simulink model "Nghich_luu2"  (R2019a)
settings: Solver=VariableStepAuto  StartTime=0.0  StopTime=10.0  RelTol=1e-3
libraries: powerlib x17, powerlib_meascontrol x2
settings Model: Creator=Admin  LastModifiedBy=Admin

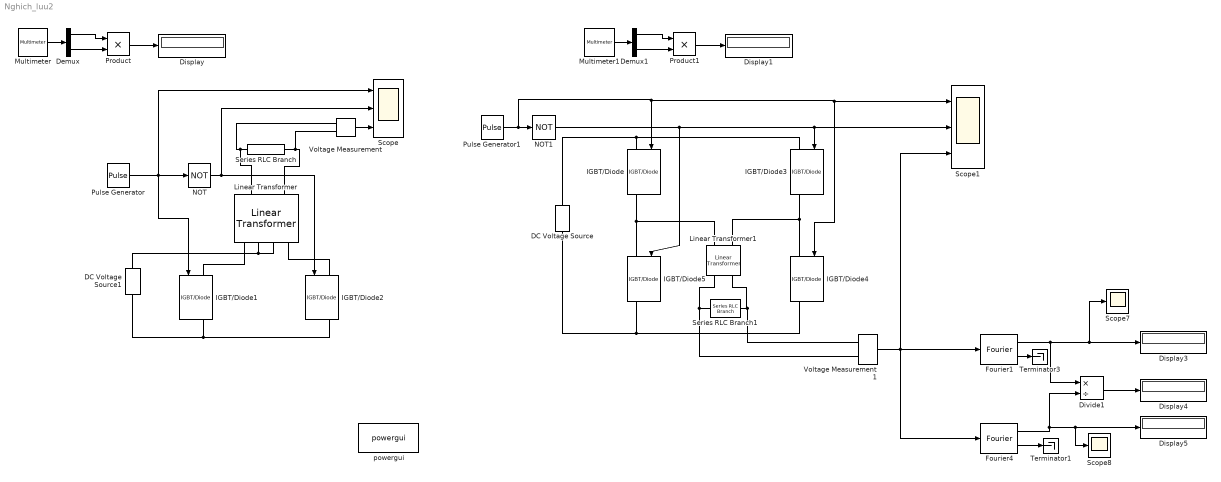
== system Nghich_luu2 ==
  DC Voltage Source : powerlib/Electrical Sources/DC Voltage Source  Amplitude=100  Measurements=None
      settings: SourceProductName=Simscape Electrical
  DC Voltage Source1 : powerlib/Electrical Sources/DC Voltage Source  Amplitude=12  Measurements=None
      settings: SourceProductName=Simscape Electrical
  Demux : Demux  Outputs=2
  Demux1 : Demux  Outputs=2
  Display{,1,3..5} (5 alike) : Display
  Divide1 : Product  Inputs=*/
  Fourier1 : powerlib_meascontrol/Measurements/Fourier  Freq=50  n=1  InInit=[0, 0]  Ts=0
      settings: SourceProductName=Simscape Electrical
  Fourier4 : powerlib_meascontrol/Measurements/Fourier  Freq=50  n=0  InInit=[0, 0]  Ts=0
      settings: SourceProductName=Simscape Electrical
  IGBT/Diode{,1..5} (6 alike) : powerlib/Power Electronics/IGBT//Diode  Ron=1e-3  Rs=1e5  Cs=inf  Measurements=on
      settings: SourceProductName=Simscape Electrical
  Linear Transformer : powerlib/Elements/Linear Transformer  UNITS=SI  NominalPower=[200 50]  winding1=[220 0 0]  winding2=[12 0 0]  ThreeWindings=on  winding3=[12 0 0]  RmLm=[1.21e+05 385.15]  Measurements=None  DataType=on
      settings: SourceProductName=Simscape Electrical
  Linear Transformer1 : powerlib/Elements/Linear Transformer  UNITS=SI  NominalPower=[ 300 50 ]  winding1=[12 0.02 0]  winding2=[220 0.05 0]  ThreeWindings=off  winding3=[3.15e+05 0.7938 0.084224]  RmLm=[inf inf]  Measurements=None  DataType=on
      settings: SourceProductName=Simscape Electrical
  Multimeter : powerlib/Measurements/Multimeter  PhasorSimulation=off  OutputType=Complex  sel=[1 3]  L=4  Gain=[1 1]  yselected={'Ub: Series RLC Branch','Ib: Series RLC Branch'};  PSBOutputType=1  PSBequivalent=0  AxesSetting=[0,0.1,-100,100]  Display=0  SavedBlockNames=-11
      settings: SourceProductName=Simscape Electrical
  Multimeter1 : powerlib/Measurements/Multimeter  PhasorSimulation=off  OutputType=Complex  sel=[2 4]  L=4  Gain=[1 1]  yselected={'Ub: Series RLC Branch1','Ib: Series RLC Branch1'};  PSBOutputType=1  PSBequivalent=0  AxesSetting=[0,0.1,-100,100]  Display=0  SavedBlockNames=-11
      settings: SourceProductName=Simscape Electrical
  NOT : Logic  Operator=NOT  IconShape=distinctive  AllPortsSameDT=off  OutDataTypeStr=boolean
  NOT1 : Logic  Operator=NOT  IconShape=distinctive  AllPortsSameDT=off  OutDataTypeStr=boolean
  Product : Product
  Product1 : Product
  Pulse Generator : DiscretePulseGenerator  PulseType=Time based  Period=0.02  PulseWidth=50
  Pulse Generator1 : DiscretePulseGenerator  PulseType=Time based  Period=0.02  PulseWidth=50
  Scope : Scope  NumInputPorts=3
  Scope1 : Scope  NumInputPorts=3
  Scope7 : Scope
  Scope8 : Scope
  Series RLC Branch : powerlib/Elements/Series RLC Branch  LConnTagsString=__new0  RConnTagsString=__new0  BranchType=R  Resistance=200  Inductance=1e-3  SetiL0=off  InitialCurrent=0  Capacitance=1e-6  Setx0=off  InitialVoltage=0  Measurements=Branch voltage and current
      settings: SourceProductName=Simscape Electrical
  Series RLC Branch1 : powerlib/Elements/Series RLC Branch  LConnTagsString=__new0  RConnTagsString=__new0  BranchType=R  Resistance=1.1  Inductance=1e-3  SetiL0=off  InitialCurrent=0  Capacitance=1e-6  Setx0=off  InitialVoltage=0  Measurements=Branch voltage and current
      settings: SourceProductName=Simscape Electrical
  Terminator1 : Terminator
  Terminator3 : Terminator
  Voltage Measurement : powerlib/Measurements/Voltage Measurement  PhasorSimulation=off  OutputType=Complex  PSBequivalent=0
      settings: SourceProductName=Simscape Electrical
  Voltage Measurement1 : powerlib/Measurements/Voltage Measurement  PhasorSimulation=off  OutputType=Complex  PSBequivalent=0
      settings: SourceProductName=Simscape Electrical
  powergui : powerlib/powergui  Priority=1  SimulationMode=Continuous  SampleTime=50e-6  frequency=60  Iterations=50  frequencyindice=0  Pbase=100e6  ErrMax=1e-4  UnitsV=kV  UnitsW=MW  buscounter=0  FunctionMessages=off  echomessages=off  EnableUseOfTLC=off  CurrentSourceSwitches=off  DisableSnubberDevices=off  DisableRonSwitches=off  DisableVfSwitches=off  DisplayEquations=off  AutomaticDiscreteSolvers=off  SolverType=Tustin/Backward Euler (TBE)  Interpol=off  ExternalGateDelay=off  methode=off  Ts=100  x0status=blocks  SPID=on  SwTol=0  HookPort=off  NonlinearTolerance=0  nMaxIteration=15  ContinueOnMaxIteration=off  RestoreLinks=warning  ResistiveCurrentMeasurement=off  Frange=[0:2:500]  Ylog=off  Xlog=on  ShowGrid=off  save=off  variable=ZData  structure=0  ZoomFFT=off  StartTime=0.0  cycles=1  DisplayStyle=1  fundamental=60  FreqAxis=off  MaxFrequency=1000  frequencyindicesteady=1  RmsSteady=1  display=off
      settings: SourceProductName=Simscape Electrical
  wires:
  Voltage Measurement/1 -> Scope/3
  Pulse Generator/1 -> Scope/1, IGBT/Diode1/1, NOT/1
  NOT/1 -> Scope/2, IGBT/Diode2/1
  Pulse Generator1/1 -> IGBT/Diode4/1, Scope1/1, IGBT/Diode/1, NOT1/1
  NOT1/1 -> IGBT/Diode5/1, IGBT/Diode3/1, Scope1/2
  Fourier1/2 -> Terminator3/1
  Divide1/1 -> Display4/1
  Fourier1/1 -> Divide1/1, Scope7/1, Display3/1
  Fourier4/2 -> Terminator1/1
  Fourier4/1 -> Scope8/1, Display5/1, Divide1/2
  Voltage Measurement1/1 -> Fourier1/1, Fourier4/1, Scope1/3
  Multimeter/1 -> Demux/1
  Demux/1 -> Product/1
  Demux/2 -> Product/2
  Product/1 -> Display/1
  Multimeter1/1 -> Demux1/1
  Demux1/1 -> Product1/1
  Demux1/2 -> Product1/2
  Product1/1 -> Display1/1
  connections:
  DC Voltage Source1/LConn1 -- IGBT/Diode1/RConn1 -- IGBT/Diode2/RConn1
  Linear Transformer/LConn2 -- Voltage Measurement/LConn1 -- Series RLC Branch/LConn1
  Linear Transformer/RConn3 -- Linear Transformer/RConn2 -- DC Voltage Source1/RConn1
  Series RLC Branch/RConn1 -- Linear Transformer/LConn1 -- Voltage Measurement/LConn2
  Linear Transformer/RConn1 -- IGBT/Diode2/LConn1
  Linear Transformer/RConn4 -- IGBT/Diode1/LConn1
  Linear Transformer1/RConn1 -- Voltage Measurement1/LConn1 -- Series RLC Branch1/RConn1
  Linear Transformer1/RConn2 -- Voltage Measurement1/LConn2 -- Series RLC Branch1/LConn1
  DC Voltage Source/RConn1 -- IGBT/Diode3/LConn1 -- IGBT/Diode/LConn1
  IGBT/Diode5/RConn1 -- DC Voltage Source/LConn1 -- IGBT/Diode4/RConn1
  IGBT/Diode/RConn1 -- Linear Transformer1/LConn2 -- IGBT/Diode5/LConn1
  IGBT/Diode3/RConn1 -- Linear Transformer1/LConn1 -- IGBT/Diode4/LConn1
